simulink model "MSFartoystyring_2_7"  (R2017b)
settings: Solver=ode45  StartTime=tstart  StopTime=tstop  RelTol=1e-3  EnableMultiTasking=on
values from neighbouring files (symbols this model uses):
  c = 1    [run_task_2_7.m]
  e_u_limit = 0.7    [run_task_2_7.m]
  Ki_u = 0.08    [run_task_2_7.m]
  Kp_los = 1/Delta    (= 0.000328083989501)    [run_task_2_7.m]
  Kp_u = 80    [run_task_2_7.m]
  omega_n_u = 0.005    [run_task_2_7.m]
  omega_psi = 0.035    [run_task_2_7.m]
  p0 = [1500 500]'    [run_task_2_7.m]
  psi0 = 50*deg2rad    (= 0.872664625997)    [run_task_2_7.m]
  r0 = 0    [run_task_2_7.m]
  tsamp = 100    [run_task_2_7.m]
  U_max = 7    [run_task_2_7.m]
  U_target = 3    [run_task_2_7.m]
  v0 = [6.63 0]'    [run_task_2_7.m]
  wp = wp.WP    [run_task_2_7.m]
  zeta = 1    [run_task_2_7.m]
  zeta_u = 1    [run_task_2_7.m]
undefined symbols (not defined in the file or in its folder): Kd_psi, Ki_psi, Ki_r, Kp_psi, Kp_r, msfartoystyring
settings Model: ExtModeAutoUpdateStatusClock=off  Creator=christh  LastModifiedBy=EllaLovise
settings DataIOCC: LimitDataPoints=on  SaveFormat=Array  SignalLoggingSaveFormat=ModelDataLogs
settings OptimizationCC: ExpressionDepthLimit=2147483647  InitFltsAndDblsToZero=on  LifeSpan=inf
settings DebuggingCC: UnderspecifiedInitializationDetection=Classic  MergeDetectMultiDrivingBlocksExec=none  SolverPrmCheckMsg=warning  FcnCallInpInsideContextMsg=warning  StateNameClashWarn=warning  SFUnexpectedBacktrackingDiag=warning  SFNoUnconditionalDefaultTransitionDiag=warning  SFExecutionAtInitializationDiag=none
settings HardwareCC: ProdBitPerPointer=32  ProdBitPerSizeT=32  ProdBitPerPtrDiffT=32  ProdLargestAtomicFloat=None  ProdIntDivRoundTo=Undefined  ProdEndianess=Unspecified  ProdWordSize=32  ProdHWDeviceType=32-bit Generic
settings ModelReferenceCC: PropagateSignalLabelsOutOfModel=off
settings CodeAppCC: StateflowObjectComments=on
settings GRTTargetCC: TargetLangStandard=C89/C90 (ANSI)  GeneratePreprocessorConditionals=Disable all  CombineOutputUpdateFcns=off  GRTInterface=on
settings ConfigComp: CovMetricSettings=dw  CovHtmlReporting=on  CovSaveCumulativeToWorkspaceVar=on  CovSaveSingleToWorkspaceVar=on  CovExternalEMLEnable=off

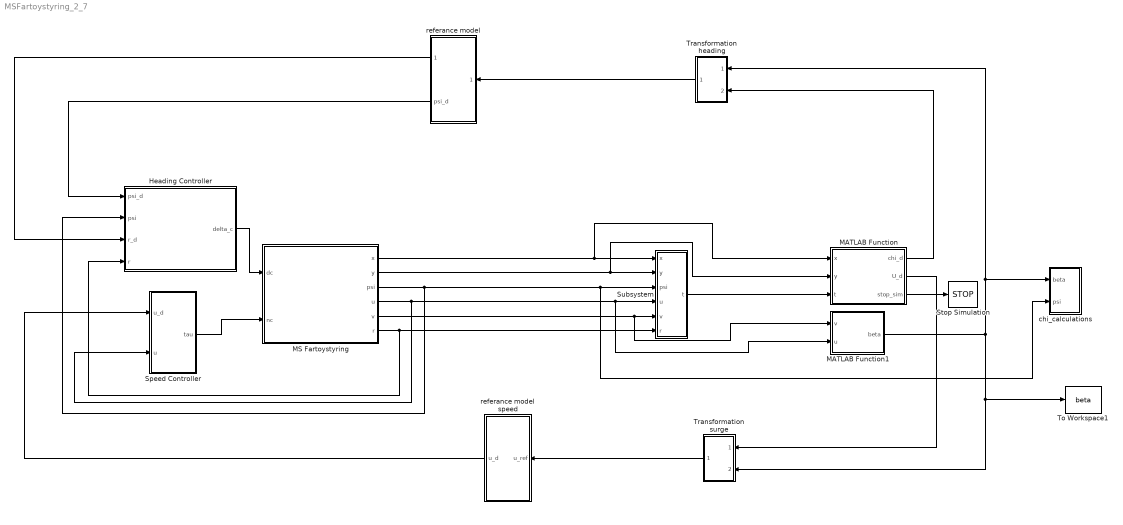
== system MSFartoystyring_2_7 ==
  Heading Controller : Subsystem
  MATLAB Function : MATLAB Function  TreatAsAtomicUnit=on
  MATLAB Function1 : MATLAB Function  TreatAsAtomicUnit=on
  MS Fartoystyring : Subsystem  mask(MS Fartoystyring for Assignment 3 G&C){x0=p0(1), y0=p0(2), u0=v0(1), v0=v0(2), psi0=psi0, r0=r0, c=c}
      mask prompts: x0 "x(t0) (m)"; y0 "y(t0) (m)"; u0 "u(t0) (m/s)"; v0 "v(t0) (m/s)"; psi0 "psi(t0) (rad)"; r0 "r(t0) (rad/s)"; c "current (0 or 1)"
      mask help:
      | Block corresponding to Figure 1 in the assignment text. Gives the response of the ship.
      |
      | The design speed of MS Fartoystyring is u=8.23 m/s.
      |
      | Input:
      | dc: commanded rudder (rad), dmax=25*pi/180
      | nc: commanded shaft speed (rad/s), nmax=85*2*pi/60
      |
      | Output:
      | x: north pos (m)
      | y: east pos (m)
      | u: surge (m/s)
      | v: sway (m/s)
      | psi: heading (rad)
      | r: yaw (rad/s)
      mask Help: Comments, bugs and help requests can be directed to the TA. Email on course website.
  Speed Controller : Subsystem
  Stop Simulation : Stop
  Subsystem : Subsystem
  To Workspace1 : ToWorkspace  VariableName=beta  SampleTime=tsamp
  Transformation heading : Subsystem
  Transformation surge : Subsystem
  chi_calculations : Subsystem
  referance model : Subsystem
  referance model speed : Subsystem
  wires:
  MS Fartoystyring/1(x) -> MATLAB Function/1(x), Subsystem/1(x)
  MS Fartoystyring/2(y) -> MATLAB Function/2(y), Subsystem/2(y)
  MS Fartoystyring/4(u) -> Speed Controller/2(u), MATLAB Function1/2(u), Subsystem/4(u)
  MS Fartoystyring/5(v) -> MATLAB Function1/1(v), Subsystem/5(v)
  MS Fartoystyring/6(r) -> Subsystem/6(r), Heading Controller/4(r)
  Heading Controller/1(delta_c) -> MS Fartoystyring/1(dc)
  MATLAB Function/3(stop_sim) -> Stop Simulation/1
  MATLAB Function1/1(beta) -> Transformation surge/2(beta), To Workspace1/1, chi_calculations/1(beta), Transformation heading/1(beta)
  MS Fartoystyring/3(psi) -> chi_calculations/2(psi), Subsystem/3(psi), Heading Controller/2(psi)
  Speed Controller/1(tau) -> MS Fartoystyring/2(nc)
  referance model/1(psi_d_dot) -> Heading Controller/3(r_d)
  referance model/2(psi_d) -> Heading Controller/1("psi_d ")
  Subsystem/1(t) -> MATLAB Function/3(t)
  MATLAB Function/2(U_d) -> Transformation surge/1(U_d)
  Transformation heading/1(psi_d) -> referance model/1(psi_ref)
  MATLAB Function/1(chi_d) -> Transformation heading/2(chi_d)
  Transformation surge/1(u_d) -> referance model speed/1(u_ref)
  referance model speed/1(u_d) -> Speed Controller/1(u_d)

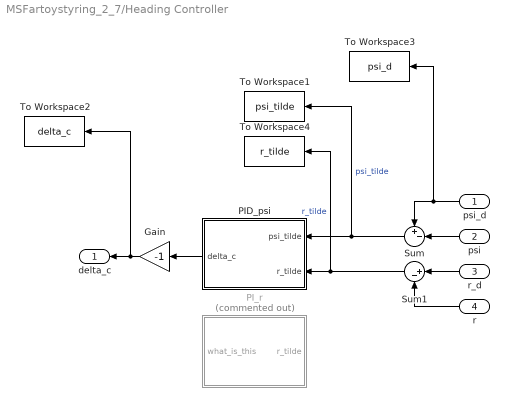
== system MSFartoystyring_2_7/Heading Controller ==
  "psi_d " : Inport
  psi : Inport  Port=2
  r_d : Inport  Port=3
  r : Inport  Port=4
  Gain : Gain  Gain=-1
  PID_psi : Subsystem
  PI_r : Subsystem  Commented=on
  Sum : Sum  Inputs=+-|
  Sum1 : Sum  Inputs=|+-
  To Workspace1 : ToWorkspace  VariableName=psi_tilde  SampleTime=tsamp
  To Workspace2 : ToWorkspace  VariableName=delta_c  SampleTime=tsamp
  To Workspace3 : ToWorkspace  VariableName=psi_d  SampleTime=tsamp
  To Workspace4 : ToWorkspace  VariableName=r_tilde  SampleTime=tsamp
  delta_c : Outport
  wires:
  psi/1 -> Sum/2
  "psi_d "/1 -> To Workspace3/1, Sum/1
  Sum1/1 -> To Workspace4/1, PID_psi/2(r_tilde)  "r_tilde"
  r_d/1 -> Sum1/1
  Sum/1 -> To Workspace1/1, PID_psi/1(psi_tilde)  "psi_tilde"
  r/1 -> Sum1/2
  Gain/1 -> To Workspace2/1, delta_c/1
  PID_psi/1(delta_c) -> Gain/1

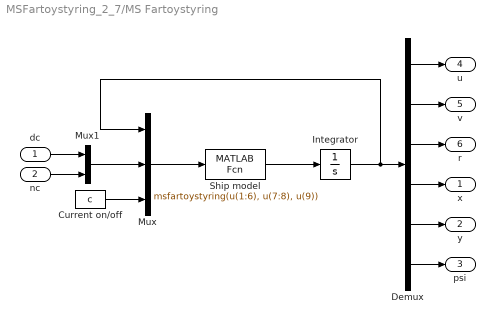
== system MSFartoystyring_2_7/MS Fartoystyring ==
  dc : Inport
  nc : Inport  Port=2
  Current on/off : Constant  Value=c
  Demux : Demux  Outputs=6
  Integrator : Integrator  InitialCondition=[u0 v0 r0 x0 y0 psi0]'
  Mux : Mux  Inputs=3
  Mux1 : Mux  Inputs=2
  Ship model : MATLABFcn  MATLABFcn=msfartoystyring(u(1:6), u(7:8), u(9))  OutputDimensions=6
  x : Outport
  y : Outport  Port=2
  psi : Outport  Port=3
  u : Outport  Port=4
  v : Outport  Port=5
  r : Outport  Port=6
  wires:
  Integrator/1 -> Mux/1, Demux/1
  Mux1/1 -> Mux/2
  dc/1 -> Mux1/1
  nc/1 -> Mux1/2
  Demux/1 -> u/1
  Demux/2 -> v/1
  Demux/3 -> r/1
  Demux/4 -> x/1
  Demux/5 -> y/1
  Demux/6 -> psi/1
  Current on/off/1 -> Mux/3
  Ship model/1 -> Integrator/1
  Mux/1 -> Ship model/1

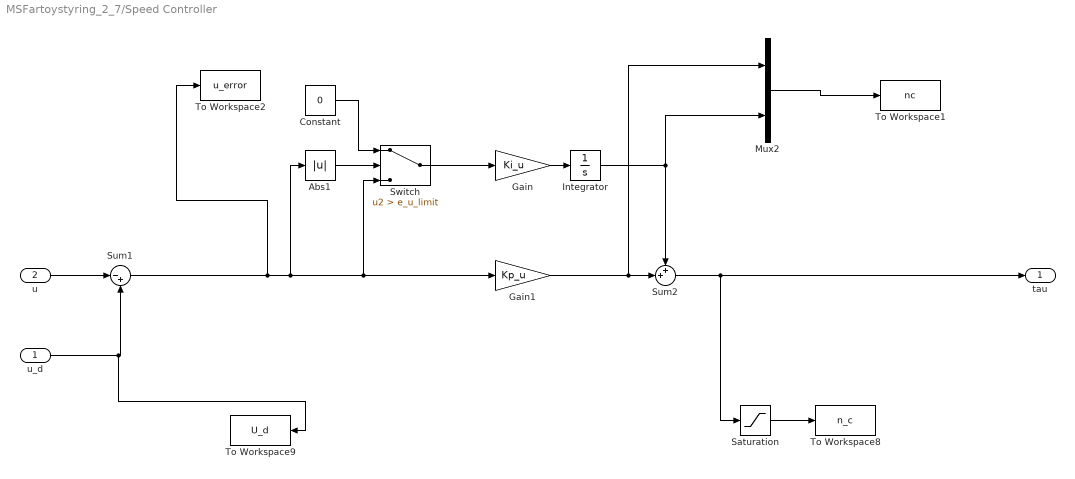
== system MSFartoystyring_2_7/Speed Controller ==
  u_d : Inport
  u : Inport  Port=2
  Abs1 : Abs
  Constant : Constant  Value=0
  Gain : Gain  Gain=Ki_u
  Gain1 : Gain  Gain=Kp_u
  Integrator : Integrator
  Mux2 : Mux  Inputs=2
  Saturation : Saturate  UpperLimit=85*2*pi/60  LowerLimit=-85*2*pi/60
  Sum1 : Sum  Inputs=|-+
  Sum2 : Sum  Inputs=++|
  Switch : Switch  Criteria=u2 > Threshold  Threshold=e_u_limit
  To Workspace1 : ToWorkspace  VariableName=nc  SampleTime=tsamp
  To Workspace2 : ToWorkspace  VariableName=u_error  SaveFormat=Structure With Time  SampleTime=tsamp
  To Workspace8 : ToWorkspace  VariableName=n_c  SampleTime=tsamp
  To Workspace9 : ToWorkspace  VariableName=U_d  SampleTime=tsamp
  tau : Outport
  wires:
  Gain/1 -> Integrator/1
  Mux2/1 -> To Workspace1/1
  Abs1/1 -> Switch/2
  Constant/1 -> Switch/1
  Switch/1 -> Gain/1
  Gain1/1 -> Mux2/1, Sum2/2
  Integrator/1 -> Mux2/2, Sum2/1
  u/1 -> Sum1/1
  u_d/1 -> To Workspace9/1, Sum1/2
  Sum2/1 -> Saturation/1, tau/1
  Sum1/1 -> To Workspace2/1, Switch/3, Gain1/1, Abs1/1
  Saturation/1 -> To Workspace8/1

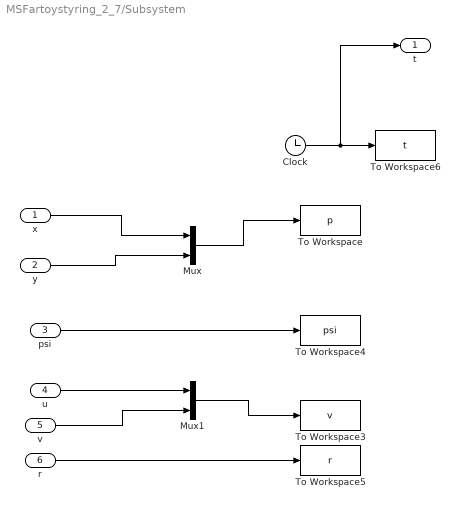
== system MSFartoystyring_2_7/Subsystem ==
  x : Inport
  y : Inport  Port=2
  psi : Inport  Port=3
  u : Inport  Port=4
  v : Inport  Port=5
  r : Inport  Port=6
  Clock : Clock
  Mux : Mux  Inputs=2
  Mux1 : Mux  Inputs=2
  To Workspace : ToWorkspace  VariableName=p  SampleTime=tsamp
  To Workspace3 : ToWorkspace  VariableName=v  SampleTime=tsamp
  To Workspace4 : ToWorkspace  VariableName=psi  SampleTime=tsamp
  To Workspace5 : ToWorkspace  VariableName=r  SampleTime=tsamp
  To Workspace6 : ToWorkspace  VariableName=t  SampleTime=tsamp
  t : Outport
  wires:
  y/1 -> Mux/2
  u/1 -> Mux1/1
  v/1 -> Mux1/2
  x/1 -> Mux/1
  r/1 -> To Workspace5/1
  psi/1 -> To Workspace4/1
  Mux/1 -> To Workspace/1
  Clock/1 -> t/1, To Workspace6/1
  Mux1/1 -> To Workspace3/1

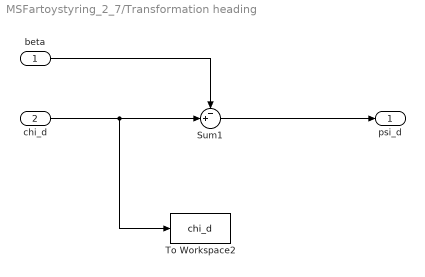
== system MSFartoystyring_2_7/Transformation heading ==
  beta : Inport
  chi_d : Inport  Port=2
  Sum1 : Sum  Inputs=-+|
  To Workspace2 : ToWorkspace  VariableName=chi_d  SampleTime=tsamp
  psi_d : Outport
  wires:
  Sum1/1 -> psi_d/1
  chi_d/1 -> To Workspace2/1, Sum1/2
  beta/1 -> Sum1/1

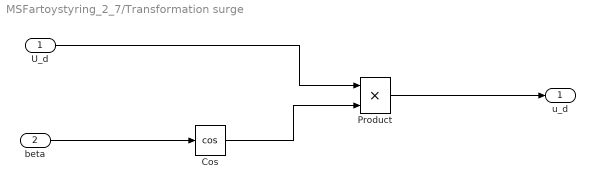
== system MSFartoystyring_2_7/Transformation surge ==
  U_d : Inport
  beta : Inport  Port=2
  Cos : Trigonometry  Operator=cos
  Product : Product
  u_d : Outport
  wires:
  Product/1 -> u_d/1
  Cos/1 -> Product/2
  U_d/1 -> Product/1
  beta/1 -> Cos/1

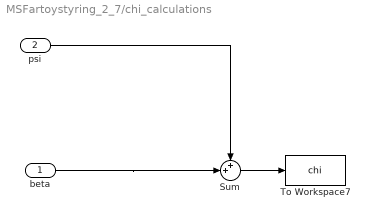
== system MSFartoystyring_2_7/chi_calculations ==
  beta : Inport
  psi : Inport  Port=2
  Sum : Sum  Inputs=++|
  To Workspace7 : ToWorkspace  VariableName=chi  SampleTime=tsamp
  wires:
  Sum/1 -> To Workspace7/1
  beta/1 -> Sum/2
  psi/1 -> Sum/1

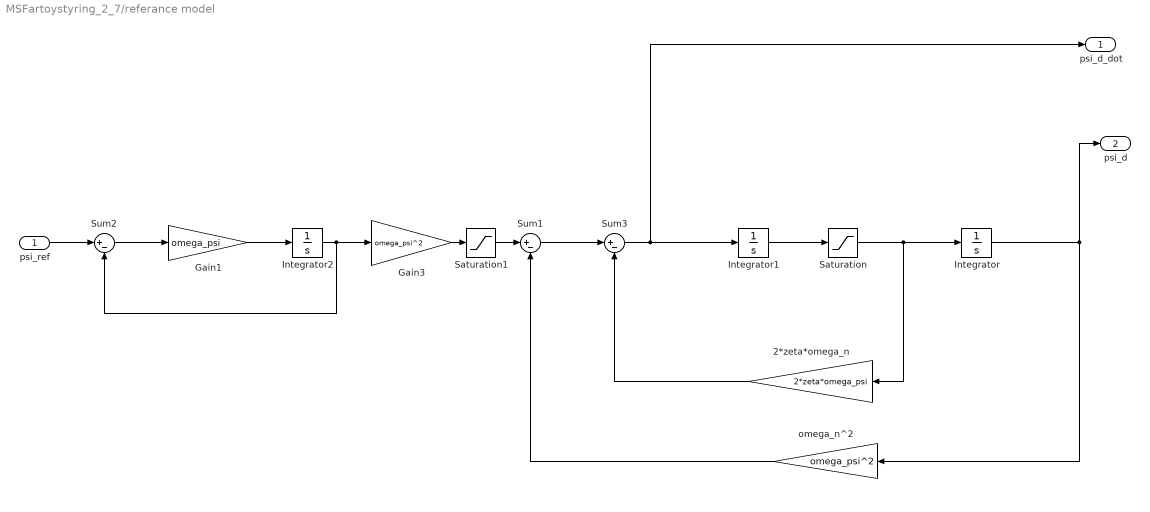
== system MSFartoystyring_2_7/referance model ==
  psi_ref : Inport
  2*zeta*omega_n : Gain  Gain=2*zeta*omega_psi
  Gain1 : Gain  Gain=omega_psi
  Gain3 : Gain  Gain=omega_psi^2
  Integrator : Integrator
  Integrator1 : Integrator
  Integrator2 : Integrator
  Saturation : Saturate  UpperLimit=100  LowerLimit=-100
  Saturation1 : Saturate  UpperLimit=100  LowerLimit=-100
  Sum1 : Sum  Inputs=|+-
  Sum2 : Sum  Inputs=|+-
  Sum3 : Sum  Inputs=|+-
  omega_n^2 : Gain  Gain=omega_psi^2
  psi_d_dot : Outport
  psi_d : Outport  Port=2
  wires:
  2*zeta*omega_n/1 -> Sum3/2
  omega_n^2/1 -> Sum1/2
  Sum3/1 -> psi_d_dot/1, Integrator1/1
  Sum1/1 -> Sum3/1
  Integrator1/1 -> Saturation/1
  Gain1/1 -> Integrator2/1
  Integrator2/1 -> Sum2/2, Gain3/1
  Sum2/1 -> Gain1/1
  psi_ref/1 -> Sum2/1
  Integrator/1 -> psi_d/1, omega_n^2/1
  Saturation/1 -> 2*zeta*omega_n/1, Integrator/1
  Saturation1/1 -> Sum1/1
  Gain3/1 -> Saturation1/1

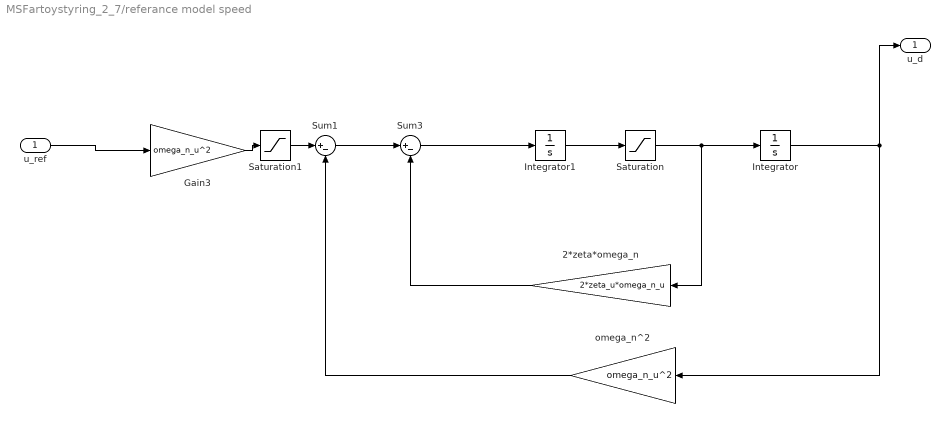
== system MSFartoystyring_2_7/referance model speed ==
  u_ref : Inport
  2*zeta*omega_n : Gain  Gain=2*zeta_u*omega_n_u
  Gain3 : Gain  Gain=omega_n_u^2
  Integrator : Integrator
  Integrator1 : Integrator
  Saturation : Saturate  UpperLimit=100  LowerLimit=-100
  Saturation1 : Saturate  UpperLimit=100  LowerLimit=-100
  Sum1 : Sum  Inputs=|+-
  Sum3 : Sum  Inputs=|+-
  omega_n^2 : Gain  Gain=omega_n_u^2
  u_d : Outport
  wires:
  2*zeta*omega_n/1 -> Sum3/2
  omega_n^2/1 -> Sum1/2
  Sum3/1 -> Integrator1/1
  Sum1/1 -> Sum3/1
  Integrator1/1 -> Saturation/1
  Integrator/1 -> u_d/1, omega_n^2/1
  Saturation/1 -> 2*zeta*omega_n/1, Integrator/1
  Saturation1/1 -> Sum1/1
  Gain3/1 -> Saturation1/1
  u_ref/1 -> Gain3/1

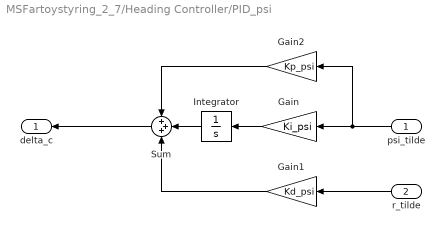
== system MSFartoystyring_2_7/Heading Controller/PID_psi ==
  psi_tilde : Inport
  r_tilde : Inport  Port=2
  Gain : Gain  Gain=Ki_psi
  Gain1 : Gain  Gain=Kd_psi
  Gain2 : Gain  Gain=Kp_psi
  Integrator : Integrator
  Sum : Sum  Inputs=+++
  delta_c : Outport
  wires:
  Gain2/1 -> Sum/1
  r_tilde/1 -> Gain1/1
  Gain1/1 -> Sum/3
  psi_tilde/1 -> Gain2/1, Gain/1
  Sum/1 -> delta_c/1
  Gain/1 -> Integrator/1
  Integrator/1 -> Sum/2

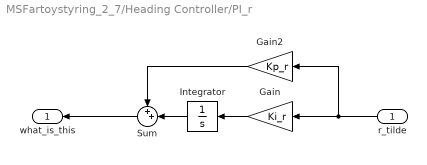
== system MSFartoystyring_2_7/Heading Controller/PI_r ==
  r_tilde : Inport
  Gain : Gain  Gain=Ki_r
  Gain2 : Gain  Gain=Kp_r
  Integrator : Integrator
  Sum : Sum  Inputs=++|
  what_is_this : Outport
  wires:
  Gain2/1 -> Sum/1
  r_tilde/1 -> Gain2/1, Gain/1
  Sum/1 -> what_is_this/1
  Gain/1 -> Integrator/1
  Integrator/1 -> Sum/2

== matlab function MSFartoystyring_2_7/MATLAB Function1 ==
  data: v input; u input; beta output
function beta = fcn(v, u)

beta = atan2(v,u);

end

== matlab function MSFartoystyring_2_7/MATLAB Function ==
  settings: updateMethod=DISCRETE  sampleTime=1
  data: chi_d output; U_d output; x input; y input; Kp_los parameter; U_target parameter; t input; wp parameter; stop_sim output; U_max parameter
function [chi_d, U_d, stop_sim] = fcn(x, y, Kp_los, U_target, t, wp, U_max)

persistent epsilon
persistent sum_dist_err
persistent prev_dist_err

% Initialization
R = 500;
if isempty(epsilon)
    Delta = 3000;
	epsilon = zeros(2,1);
else
    Delta = sqrt(abs(R^2 - epsilon(2)^2));
end
Kp = 1/Delta;
    
if isempty(sum_dist_err)
    sum_dist_err = 0;
end
if isempty(prev_dist_err)
    prev_dist_err = 0;
end

%%%%%%%%%%%%%%%%%%%%%%%%%%%%%%%%%%%%%%%

stop_sim = 0;

% Get unit direction of target ship
target_vec = (wp(:,2)-wp(:,1))./norm(wp(:,2)-wp(:,1)); %unit vector
% our position
p_b = [x y]';

% Get current waypoints
p_wp1 = wp(:,2);     % Targets start position is our initial position
p_wp2 = p_wp1 + target_vec.*U_target.*t - 350.*target_vec;


% Calculate chi_d
alpha = atan2(p_wp2(2)-p_wp1(2), p_wp2(1) - p_wp1(1));

Rp = [cos(alpha) -sin(alpha);
      sin(alpha) cos(alpha) ];
epsilon = Rp'*(p_b - p_wp1);
chi_d = mod(alpha + atan(-Kp_los*epsilon(2)), 2*pi);

%%%%%%%%%%%%%%%%%%%%%%%%%%%%%%%%%%%%%%%%%%%%%%%%%%%%%%%%%%%%%%%%

% Calculate desired speed
sign = 1;
if (norm(p_b - p_wp1) > norm(p_wp2 - p_wp1))
    sign = -1;
end

Kp_speed = 0.01;
Ki_speed = 1*10^(-5);
Kd_speed = 5;

dist_err = norm(p_wp2 - p_b)*sign;

if (abs(dist_err) < 400)
    sum_dist_err = sum_dist_err + dist_err;
end

der_err = dist_err - prev_dist_err;

controller_val = Kp_speed*(dist_err) + Ki_speed*sum_dist_err + Kd_speed*der_err;


%U_d = U_target + min(U_max-U_target, max(-U_target + 1, controller_val)); %U_target + (U_max-U_target)*(1-1/norm(p_wp1 - p_wp2)); %U_target - U_max*epsilon(2)/sqrt(epsilon(2)^2 + Delta_s^2);
p_tilde = p_b - p_wp2;
delta_p = 5600;
if(norm(p_tilde) >2500 )
    delta_p = 1000;
end
kapa = (7 - U_target)*norm(p_tilde)/sqrt(p_tilde'*p_tilde + delta_p^2);
v_t = [U_target*cos(alpha); U_target*sin(alpha)];
v_a = -kapa*p_tilde/norm(p_tilde);
v_d = v_t + v_a;
U_d = norm(v_d); % ned position

prev_dist_err = dist_err;
end
